simulink model "sampleModel1909"  (R2023a)
settings: Solver=VariableStepAuto  StartTime=0.0  StopTime=10.0  RelTol=1e-3
libraries: hdlsllib x6, simulink x2
settings Model: Creator=user1  LastModifiedBy=user1

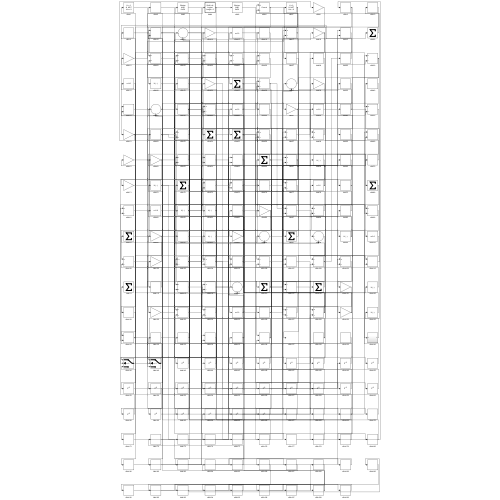
[thumbnail: Simulink's stored preview of the top-level diagram]
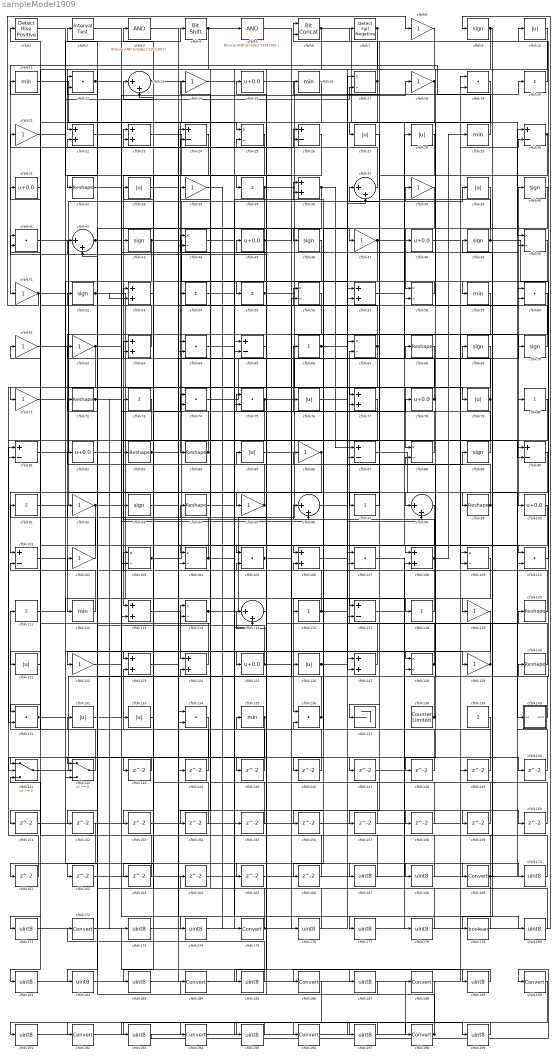
== system sampleModel1909 ==
  cfblk1 : hdlsllib/Logic and Bit Operations/Detect Rise Positive  vinit=0  OutDataTypeStr=boolean
  cfblk{10,27..28,33,39,76,79,85,121,126,132..133} (12 alike) : Abs  SaturateOnIntegerOverflow=off
  cfblk{15,31,45,48,78,82,100,125} (8 alike) : Bias  Bias=0.0  SaturateOnIntegerOverflow=off
  cfblk{24,26,30,65,81,87,90,101,117} (9 alike) : Sum  Inputs=+-
  cfblk{8,14,18,21,34,38,47,51,61..62,71,86,92,95,102,119,122,129} (18 alike) : Gain
  cfblk{17,25,44,50,56,58,67,88,103..104,109,114,128} (13 alike) : Product  Inputs=*/  RndMeth=Zero  SaturateOnIntegerOverflow=on
  cfblk{12,19,41,60,64,74..75,105,107,110,131,134,136} (13 alike) : DotProduct  OutDataTypeStr=Inherit: Inherit via internal rule
  cfblk{22..23,36,53,57,63,77,106,108,113,123..124,127} (13 alike) : Sum
  cfblk{11,16,29,59,112,135} (6 alike) : MinMax
  cfblk{20,35,54..55,66,73,80,91,97,111,116,118} (12 alike) : Sum  Inputs=+
  cfblk{13,37,42,96,98,115} (6 alike) : Sum  Inputs=|++
  cfblk{32,68,72,83..84,94,99,120,130} (9 alike) : Reshape
  cfblk137 : Terminator
  cfblk138 : hdlsllib/Sources/Counter Limited  uplimit=7  tsamp=-1
  cfblk139 : Constant  SampleTime=-1
  cfblk140 : Subsystem
      settings: LibrarySourceBlock=|
      | hdlsllib/Ports &
      | Subsystems/Subsystem
  cfblk141 : Switch  SaturateOnIntegerOverflow=off  InputSameDT=off
  cfblk142 : Switch  SaturateOnIntegerOverflow=off  InputSameDT=off
  cfblk{143..166} (24 alike) : Delay  SampleTime=1
  cfblk{167..168,170..171,173..174,176..178,180..183,185,187,189,191,193,195,197,199} (21 alike) : DataTypeConversion  OutDataTypeStr=uint8  SaturateOnIntegerOverflow=off  RndMeth=Floor
  cfblk{169,172,175,184,186,188,190,192,194,196,198} (11 alike) : DataTypeConversion  SaturateOnIntegerOverflow=off  RndMeth=Floor
  cfblk179 : DataTypeConversion  OutDataTypeStr=boolean  SaturateOnIntegerOverflow=off  RndMeth=Floor
  cfblk2 : hdlsllib/Logic and Bit Operations/Interval Test  IntervalClosedRight=on  uplimit=0.5  IntervalClosedLeft=on  lowlimit=-0.5  OutDataTypeStr=boolean
  cfblk3 : simulink/Logic and Bit Operations/Bitwise Operator  logicop=AND  UseBitMask=on  BitMask=bin2dec('11011001')  BitMaskRealWorld=Stored Integer
      settings: LibrarySourceBlock=|
      | hdlsllib/Logic and Bit
      | Operations/Bitwise
      | Operator
  cfblk4 : hdlsllib/Logic and Bit Operations/Bit Shift  mode=Shift Left Logical  N=0
  cfblk{9,40,43,46,49,52,69..70,89,93} (10 alike) : Signum
  cfblk5 : simulink/Logic and Bit Operations/Bitwise Operator  logicop=AND  UseBitMask=on  BitMask=bin2dec('11011001')  BitMaskRealWorld=Stored Integer
      settings: LibrarySourceBlock=|
      | hdlsllib/Logic and Bit
      | Operations/Bitwise
      | Operator
  cfblk6 : hdlsllib/Logic and Bit Operations/Bit Concat  numInputs=2
  cfblk7 : hdlsllib/Logic and Bit Operations/Detect Fall Negative  vinit=0  OutDataTypeStr=boolean
  wires:
  cfblk35/1 -> cfblk100/1, cfblk142/1
  cfblk24/1 -> cfblk113/1
  cfblk130/1 -> cfblk67/2
  cfblk81/1 -> cfblk38/1
  cfblk70/1 -> cfblk22/1
  cfblk68/1 -> cfblk113/2
  cfblk41/1 -> cfblk98/1
  cfblk29/1 -> cfblk51/1
  cfblk52/1 -> cfblk136/1, cfblk53/2
  cfblk56/1 -> cfblk112/1
  cfblk15/1 -> cfblk79/1
  cfblk142/1 -> cfblk111/1
  cfblk103/1 -> cfblk39/1, cfblk105/1
  cfblk49/1 -> cfblk130/1, cfblk16/1
  cfblk87/1 -> cfblk140/1(In1)
  cfblk62/1 -> cfblk121/1, cfblk50/2
  cfblk63/1 -> cfblk52/1
  cfblk100/1 -> cfblk141/1
  cfblk72/1 -> cfblk24/2, cfblk173/1
  cfblk108/1 -> cfblk73/1, cfblk29/1, cfblk166/1
  cfblk11/1 -> cfblk84/1
  cfblk88/1 -> cfblk23/1
  cfblk125/1 -> cfblk72/1, cfblk159/1
  cfblk74/1 -> cfblk28/1
  cfblk89/1 -> cfblk66/1
  cfblk38/1 -> cfblk106/1
  cfblk13/1 -> cfblk25/1, cfblk110/2
  cfblk78/1 -> cfblk22/2, cfblk7/1
  cfblk47/1 -> cfblk123/1, cfblk110/1
  cfblk45/1 -> cfblk43/1, cfblk47/1, cfblk162/1
  cfblk133/1 -> cfblk33/1
  cfblk118/1 -> cfblk117/1
  cfblk124/1 -> cfblk11/1
  cfblk75/1 -> cfblk122/1, cfblk90/2
  cfblk92/1 -> cfblk142/3, cfblk174/1
  cfblk27/1 -> cfblk77/1
  cfblk39/1 -> cfblk58/1
  cfblk17/1 -> cfblk6/1, cfblk103/2
  cfblk51/1 -> cfblk8/1, cfblk26/2, cfblk127/2
  cfblk57/1 -> cfblk48/1
  cfblk122/1 -> cfblk18/1
  cfblk83/1 -> cfblk26/1, cfblk60/2
  cfblk10/1 -> cfblk95/1
  cfblk97/1 -> cfblk37/1
  cfblk55/1 -> cfblk80/1, cfblk90/1
  cfblk61/1 -> cfblk88/1
  cfblk127/1 -> cfblk94/1
  cfblk114/1 -> cfblk40/1, cfblk36/2
  cfblk18/1 -> cfblk27/1, cfblk58/2
  cfblk139/1 -> cfblk123/2
  cfblk6/1 -> cfblk50/1, cfblk32/1
  cfblk138/1 -> cfblk56/1, cfblk103/1
  cfblk66/1 -> cfblk98/2, cfblk156/1
  cfblk53/1 -> cfblk23/2
  cfblk113/1 -> cfblk124/1
  cfblk19/1 -> cfblk108/1
  cfblk40/1 -> cfblk137/1
  cfblk59/1 -> cfblk125/1
  cfblk4/1 -> cfblk5/1, cfblk44/2
  cfblk131/1 -> cfblk31/1, cfblk145/1
  cfblk25/1 -> cfblk64/2
  cfblk109/1 -> cfblk116/1
  cfblk20/1 -> cfblk6/2
  cfblk34/1 -> cfblk175/1
  cfblk8/1 -> cfblk54/1
  cfblk91/1 -> cfblk99/1
  cfblk37/1 -> cfblk13/2
  cfblk31/1 -> cfblk71/1
  cfblk36/1 -> cfblk83/1, cfblk87/1
  cfblk123/1 -> cfblk70/1
  cfblk28/1 -> cfblk97/1
  cfblk79/1 -> cfblk68/1, cfblk183/1
  cfblk140/1(Out1) -> cfblk88/2
  cfblk105/1 -> cfblk45/1, cfblk77/2
  cfblk106/1 -> cfblk57/1
  cfblk136/1 -> cfblk114/1, cfblk92/1
  cfblk16/1 -> cfblk131/1
  cfblk58/1 -> cfblk55/1
  cfblk9/1 -> cfblk59/1, cfblk151/1
  cfblk54/1 -> cfblk115/2
  cfblk85/1 -> cfblk19/2
  cfblk23/1 -> cfblk76/1
  cfblk44/1 -> cfblk129/1
  cfblk102/1 -> cfblk61/1
  cfblk69/1 -> cfblk126/1
  cfblk132/1 -> cfblk74/1
  cfblk104/1 -> cfblk42/2, cfblk155/1, cfblk158/1
  cfblk129/1 -> cfblk102/1, cfblk96/1
  cfblk12/1 -> cfblk46/1, cfblk87/2
  cfblk110/1 -> cfblk10/1
  cfblk99/1 -> cfblk63/1, cfblk36/1
  cfblk67/1 -> cfblk131/2, cfblk41/2, cfblk163/1
  cfblk128/1 -> cfblk21/1, cfblk41/1, cfblk82/1
  cfblk21/1 -> cfblk4/1
  cfblk60/1 -> cfblk109/2
  cfblk7/1 -> cfblk117/2, cfblk75/2
  cfblk95/1 -> cfblk42/1, cfblk62/1
  cfblk94/1 -> cfblk78/1
  cfblk115/1 -> cfblk15/1
  cfblk111/1 -> cfblk118/1
  cfblk96/1 -> cfblk89/1
  cfblk107/1 -> cfblk169/1
  cfblk86/1 -> cfblk101/1, cfblk104/2
  cfblk112/1 -> cfblk91/1
  cfblk30/1 -> cfblk128/1, cfblk179/1
  cfblk135/1 -> cfblk75/1, cfblk152/1
  cfblk48/1 -> cfblk30/2
  cfblk71/1 -> cfblk17/2
  cfblk116/1 -> cfblk101/2, cfblk69/1, cfblk37/2
  cfblk43/1 -> cfblk127/1, cfblk142/2, cfblk160/1
  cfblk1/1 -> cfblk35/1
  cfblk126/1 -> cfblk120/1, cfblk86/1
  cfblk76/1 -> cfblk20/1
  cfblk141/1 -> cfblk56/2
  cfblk42/1 -> cfblk12/1, cfblk96/2
  cfblk120/1 -> cfblk44/1
  cfblk82/1 -> cfblk93/1
  cfblk90/1 -> cfblk119/1
  cfblk73/1 -> cfblk81/2
  cfblk84/1 -> cfblk104/1, cfblk53/1
  cfblk26/1 -> cfblk143/1
  cfblk143/1 -> cfblk141/2
  cfblk33/1 -> cfblk144/1
  cfblk144/1 -> cfblk63/2
  cfblk145/1 -> cfblk64/1
  cfblk50/1 -> cfblk146/1
  cfblk146/1 -> cfblk1/1
  cfblk32/1 -> cfblk147/1
  cfblk147/1 -> cfblk108/2
  cfblk80/1 -> cfblk148/1
  cfblk148/1 -> cfblk106/2
  cfblk149/1 -> cfblk136/2
  cfblk22/1 -> cfblk150/1
  cfblk150/1 -> cfblk60/1
  cfblk151/1 -> cfblk19/1
  cfblk77/1 -> cfblk153/1
  cfblk153/1 -> cfblk109/1
  cfblk46/1 -> cfblk154/1
  cfblk154/1 -> cfblk13/1
  cfblk155/1 -> cfblk124/2
  cfblk156/1 -> cfblk17/1
  cfblk98/1 -> cfblk157/1
  cfblk157/1 -> cfblk67/1
  cfblk158/1 -> cfblk25/2
  cfblk159/1 -> cfblk74/2
  cfblk160/1 -> cfblk105/2
  cfblk121/1 -> cfblk161/1
  cfblk161/1 -> cfblk81/1
  cfblk162/1 -> cfblk57/2
  cfblk163/1 -> cfblk141/3
  cfblk164/1 -> cfblk128/2
  cfblk93/1 -> cfblk165/1
  cfblk165/1 -> cfblk30/1
  cfblk166/1 -> cfblk114/2
  cfblk2/1 -> cfblk167/1
  cfblk167/1 -> cfblk85/1
  cfblk101/1 -> cfblk168/1
  cfblk168/1 -> cfblk2/1
  cfblk169/1 -> cfblk164/1, cfblk24/1, cfblk49/1
  cfblk64/1 -> cfblk170/1
  cfblk170/1 -> cfblk107/1
  cfblk152/1 -> cfblk171/1
  cfblk171/1 -> cfblk107/2
  cfblk173/1 -> cfblk65/1
  cfblk174/1 -> cfblk65/2
  cfblk175/1 -> cfblk132/1, cfblk133/1
  cfblk5/1 -> cfblk176/1
  cfblk176/1 -> cfblk34/1
  cfblk14/1 -> cfblk177/1
  cfblk177/1 -> cfblk9/1
  cfblk117/1 -> cfblk178/1
  cfblk178/1 -> cfblk14/1
  cfblk179/1 -> cfblk3/1
  cfblk3/1 -> cfblk180/1
  cfblk180/1 -> cfblk115/1
  cfblk134/1 -> cfblk181/1
  cfblk181/1 -> cfblk149/1
  cfblk119/1 -> cfblk182/1
  cfblk182/1 -> cfblk134/1
  cfblk183/1 -> cfblk134/2
  cfblk65/1 -> cfblk185/1
  cfblk185/1 -> cfblk172/1
  cfblk172/1 -> cfblk187/1
  cfblk187/1 -> cfblk184/1
  cfblk184/1 -> cfblk189/1
  cfblk189/1 -> cfblk186/1
  cfblk186/1 -> cfblk191/1
  cfblk191/1 -> cfblk188/1
  cfblk188/1 -> cfblk193/1
  cfblk193/1 -> cfblk190/1
  cfblk190/1 -> cfblk195/1
  cfblk195/1 -> cfblk192/1
  cfblk196/1 -> cfblk198/1
  cfblk192/1 -> cfblk197/1
  cfblk197/1 -> cfblk194/1
  cfblk198/1 -> cfblk12/2, cfblk135/1
  cfblk194/1 -> cfblk199/1
  cfblk199/1 -> cfblk196/1

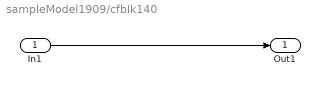
== system sampleModel1909/cfblk140 ==
  In1 : Inport
  Out1 : Outport
  wires:
  In1/1 -> Out1/1
